simulink model "Digital_Optimal_Control_HW2_1d"  (R2018b)
settings: Solver=VariableStepAuto  StartTime=0.0  StopTime=20  RelTol=1e-3
values from neighbouring files (symbols this model uses):
  h = 0.014    [Homework1.m]
libraries: simulink x1
settings Model: Creator=Janne  LastModifiedBy=Henkka

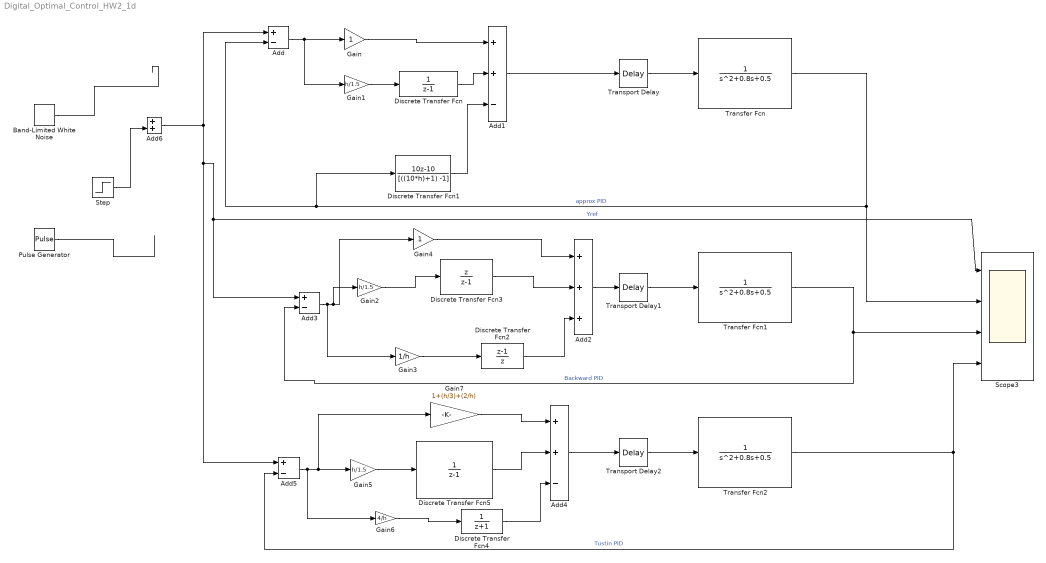
== system Digital_Optimal_Control_HW2_1d ==
  Add : Sum  Inputs=+-
  Add1 : Sum  Inputs=++-
  Add2 : Sum  Inputs=+++
  Add3 : Sum  Inputs=+-
  Add4 : Sum  Inputs=++-
  Add5 : Sum  Inputs=+-
  Add6 : Sum
  Band-Limited White Noise : simulink/Sources/Band-Limited White Noise  Cov=[0.5]  Ts=h  seed=[23341]
  Discrete Transfer Fcn : DiscreteTransferFcn  Denominator=[1 -1]  SampleTime=h
  Discrete Transfer Fcn1 : DiscreteTransferFcn  Numerator=[10 -10]  Denominator=[((10*h)+1) -1]  SampleTime=h
  Discrete Transfer Fcn2 : DiscreteTransferFcn  Numerator=[1 -1]  Denominator=[1 0]  SampleTime=h
  Discrete Transfer Fcn3 : DiscreteTransferFcn  Numerator=[1 0]  Denominator=[1 -1]  SampleTime=h
  Discrete Transfer Fcn4 : DiscreteTransferFcn  Denominator=[1 1]  SampleTime=h
  Discrete Transfer Fcn5 : DiscreteTransferFcn  Denominator=[1 -1]  SampleTime=h
  Gain : Gain
  Gain1 : Gain  Gain=h/1.5
  Gain2 : Gain  Gain=h/1.5
  Gain3 : Gain  Gain=1/h
  Gain4 : Gain
  Gain5 : Gain  Gain=h/1.5
  Gain6 : Gain  Gain=4/h
  Gain7 : Gain  Gain=1+(h/3)+(2/h)
  Pulse Generator : DiscretePulseGenerator  PulseType=Time based  Period=10  PulseWidth=5
  Scope3 : Scope  NumInputPorts=4
  Step : Step  SampleTime=0
  Transfer Fcn : TransferFcn  Denominator=[1 0.8 0.5]
  Transfer Fcn1 : TransferFcn  Denominator=[1 0.8 0.5]
  Transfer Fcn2 : TransferFcn  Denominator=[1 0.8 0.5]
  Transport Delay : TransportDelay  DelayTime=0.7
  Transport Delay1 : TransportDelay  DelayTime=0.7
  Transport Delay2 : TransportDelay  DelayTime=0.7
  wires:
  Add/1 -> Gain1/1, Gain/1
  Gain/1 -> Add1/1
  Gain1/1 -> Discrete Transfer Fcn/1
  Discrete Transfer Fcn/1 -> Add1/2
  Discrete Transfer Fcn1/1 -> Add1/3
  Transfer Fcn/1 -> Discrete Transfer Fcn1/1, Add/2, Scope3/2  "approx PID"
  Add1/1 -> Transport Delay/1
  Transport Delay1/1 -> Transfer Fcn1/1
  Add2/1 -> Transport Delay1/1
  Gain2/1 -> Discrete Transfer Fcn3/1
  Gain4/1 -> Add2/1
  Discrete Transfer Fcn3/1 -> Add2/2
  Gain3/1 -> Discrete Transfer Fcn2/1
  Discrete Transfer Fcn2/1 -> Add2/3
  Transfer Fcn1/1 -> Add3/2, Scope3/3  "Backward PID"
  Add6/1 -> Add5/1, Add3/1, Scope3/1, Add/1  "Yref"
  Add3/1 -> Gain3/1, Gain2/1, Gain4/1
  Transport Delay/1 -> Transfer Fcn/1
  Gain5/1 -> Discrete Transfer Fcn5/1
  Transfer Fcn2/1 -> Scope3/4, Add5/2  "Tustin PID"
  Gain7/1 -> Add4/1
  Discrete Transfer Fcn5/1 -> Add4/2
  Transport Delay2/1 -> Transfer Fcn2/1
  Add4/1 -> Transport Delay2/1
  Discrete Transfer Fcn4/1 -> Add4/3
  Add5/1 -> Gain6/1, Gain5/1, Gain7/1
  Gain6/1 -> Discrete Transfer Fcn4/1
  Pulse Generator/1 -> ?
  Band-Limited White Noise/1 -> ?
  Step/1 -> Add6/2
